simulink model "silnikDC_bezwladnosc_fuzzy"  (R2013b)
settings: Solver=ode3  StartTime=0.0  StopTime=1  FixedStep=100e-6  MaxStep=0.0001  RelTol=1e-3
values from neighbouring files (symbols this model uses):
  a = 0.7    [parametryDC.m]
  B = 0.002953    [parametryDC.m]
  J = 0.02215    [parametryDC.m]
  K = 1.28    [parametryDC.m]
  k1 = 1.28    [parametryDC.m]
  La = 0.1215    [parametryDC.m]
  Ra = 11.2    [parametryDC.m]
  w_de = 1/100000    (= 1e-05)    [parametryDC.m]
  w_du = 100000    [parametryDC.m]
  w_e = 1/2000    (= 0.0005)    [parametryDC.m]
  w_u = 800    [parametryDC.m]
libraries: fuzblock x3
settings Model: Creator=Siembab  LastModifiedBy=Siembab
settings SolverCC: ZeroCrossAlgorithm=Adaptive
settings DataIOCC: SignalLoggingSaveFormat=ModelDataLogs
settings OptimizationCC: ExpressionDepthLimit=2147483647
settings DebuggingCC: FcnCallInpInsideContextMsg=UseLocalSettings  StateNameClashWarn=warning
settings GRTTargetCC: CombineOutputUpdateFcns=off  GRTInterface=on

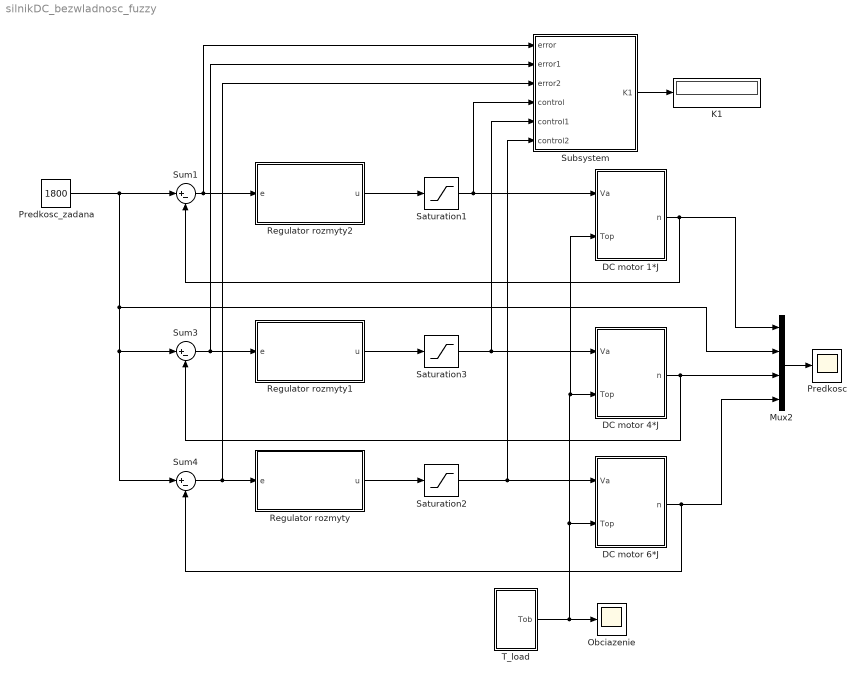
== system silnikDC_bezwladnosc_fuzzy ==
  DC motor 1*J : Subsystem
  DC motor 4*J : Subsystem
  DC motor 6*J : Subsystem
  K1 : Display
  Mux2 : Mux
  Obciazenie : Scope
      settings: TimeRange=1  YMin=1400  YMax=1825
  Predkosc : Scope
      settings: TimeRange=1  YMin=1475  YMax=1825  SaveName=ScopeData4
  Predkosc_zadana : Constant  Value=1800
  Regulator rozmyty : Subsystem
  Regulator rozmyty1 : Subsystem
  Regulator rozmyty2 : Subsystem
  Saturation1 : Saturate  UpperLimit=500  LowerLimit=-500
  Saturation2 : Saturate  UpperLimit=500  LowerLimit=-500
  Saturation3 : Saturate  UpperLimit=500  LowerLimit=-500
  Subsystem : Subsystem
  Sum1 : Sum  Inputs=|+-
  Sum3 : Sum  Inputs=|+-
  Sum4 : Sum  Inputs=|+-
  T_load : Subsystem
  wires:
  Saturation1/1 -> Subsystem/4(control), DC motor 1*J/1(Va)
  Predkosc_zadana/1 -> Sum4/1, Sum3/1, Mux2/2, Sum1/1
  DC motor 1*J/1(n) -> Sum1/2, Mux2/1
  Mux2/1 -> Predkosc/1
  DC motor 6*J/1(n) -> Sum4/2, Mux2/4
  DC motor 4*J/1(n) -> Sum3/2, Mux2/3
  Regulator rozmyty/1(u) -> Saturation2/1
  Saturation2/1 -> Subsystem/6(control2), DC motor 6*J/1(Va)
  Regulator rozmyty1/1(u) -> Saturation3/1
  Saturation3/1 -> Subsystem/5(control1), DC motor 4*J/1(Va)
  Sum3/1 -> Subsystem/2(error1), Regulator rozmyty1/1(e)
  Sum4/1 -> Subsystem/3(error2), Regulator rozmyty/1(e)
  Regulator rozmyty2/1(u) -> Saturation1/1
  Sum1/1 -> Subsystem/1(error), Regulator rozmyty2/1(e)
  T_load/1(Tob) -> Obciazenie/1, DC motor 1*J/2(Top), DC motor 4*J/2(Top), DC motor 6*J/2(Top)
  Subsystem/1(K1) -> K1/1

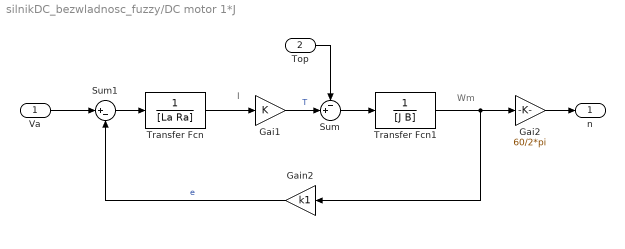
== system silnikDC_bezwladnosc_fuzzy/DC motor 1*J ==
  note: Wm
  note: I
  Va : Inport
  Top : Inport  Port=2
  Gai1 : Gain  Gain=K
  Gai2 : Gain  Gain=60/2*pi
  Gain2 : Gain  Gain=k1
  Sum : Sum  Inputs=-+|
  Sum1 : Sum  Inputs=|+-
  Transfer Fcn : TransferFcn  Denominator=[La Ra]
  Transfer Fcn1 : TransferFcn  Denominator=[J B]
  n : Outport
  wires:
  Transfer Fcn/1 -> Gai1/1
  Gai1/1 -> Sum/2  "T"
  Sum/1 -> Transfer Fcn1/1
  Gain2/1 -> Sum1/2  "e"
  Transfer Fcn1/1 -> Gai2/1, Gain2/1
  Sum1/1 -> Transfer Fcn/1
  Va/1 -> Sum1/1
  Top/1 -> Sum/1
  Gai2/1 -> n/1

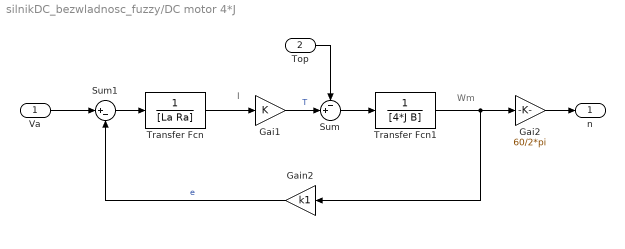
== system silnikDC_bezwladnosc_fuzzy/DC motor 4*J ==
  note: Wm
  note: I
  Va : Inport
  Top : Inport  Port=2
  Gai1 : Gain  Gain=K
  Gai2 : Gain  Gain=60/2*pi
  Gain2 : Gain  Gain=k1
  Sum : Sum  Inputs=-+|
  Sum1 : Sum  Inputs=|+-
  Transfer Fcn : TransferFcn  Denominator=[La Ra]
  Transfer Fcn1 : TransferFcn  Denominator=[4*J B]
  n : Outport
  wires:
  Transfer Fcn/1 -> Gai1/1
  Gai1/1 -> Sum/2  "T"
  Sum/1 -> Transfer Fcn1/1
  Gain2/1 -> Sum1/2  "e"
  Transfer Fcn1/1 -> Gai2/1, Gain2/1
  Sum1/1 -> Transfer Fcn/1
  Va/1 -> Sum1/1
  Top/1 -> Sum/1
  Gai2/1 -> n/1

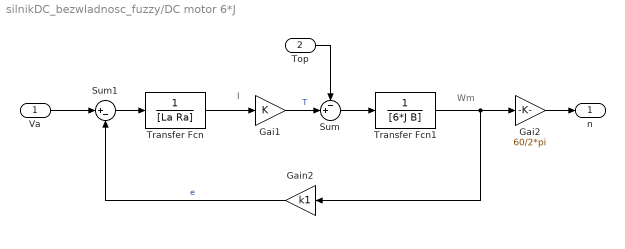
== system silnikDC_bezwladnosc_fuzzy/DC motor 6*J ==
  note: Wm
  note: I
  Va : Inport
  Top : Inport  Port=2
  Gai1 : Gain  Gain=K
  Gai2 : Gain  Gain=60/2*pi
  Gain2 : Gain  Gain=k1
  Sum : Sum  Inputs=-+|
  Sum1 : Sum  Inputs=|+-
  Transfer Fcn : TransferFcn  Denominator=[La Ra]
  Transfer Fcn1 : TransferFcn  Denominator=[6*J B]
  n : Outport
  wires:
  Transfer Fcn/1 -> Gai1/1
  Gai1/1 -> Sum/2  "T"
  Sum/1 -> Transfer Fcn1/1
  Gain2/1 -> Sum1/2  "e"
  Transfer Fcn1/1 -> Gai2/1, Gain2/1
  Sum1/1 -> Transfer Fcn/1
  Va/1 -> Sum1/1
  Top/1 -> Sum/1
  Gai2/1 -> n/1

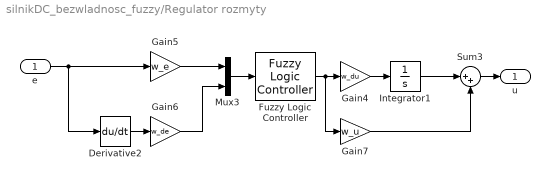
== system silnikDC_bezwladnosc_fuzzy/Regulator rozmyty ==
  e : Inport
  Derivative2 : Derivative
  Fuzzy Logic Controller : fuzblock/Fuzzy Logic  Controller  fis=RegMamdani2
  Gain4 : Gain  Gain=w_du
  Gain5 : Gain  Gain=w_e
  Gain6 : Gain  Gain=w_de
  Gain7 : Gain  Gain=w_u
  Integrator1 : Integrator
  Mux3 : Mux  Inputs=2
  Sum3 : Sum  Inputs=|++
  u : Outport
  wires:
  Derivative2/1 -> Gain6/1
  e/1 -> Derivative2/1, Gain5/1
  Sum3/1 -> u/1
  Gain6/1 -> Mux3/2
  Gain5/1 -> Mux3/1
  Gain7/1 -> Sum3/2
  Mux3/1 -> Fuzzy Logic Controller/1
  Integrator1/1 -> Sum3/1
  Gain4/1 -> Integrator1/1
  Fuzzy Logic Controller/1 -> Gain7/1, Gain4/1

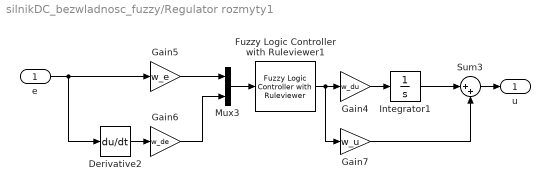
== system silnikDC_bezwladnosc_fuzzy/Regulator rozmyty1 ==
  e : Inport
  Derivative2 : Derivative
  Fuzzy Logic Controller with Ruleviewer1 : fuzblock/Fuzzy Logic  Controller  with Ruleviewer  fismatrix=RegMamdani2  Ts=0.02
  Gain4 : Gain  Gain=w_du
  Gain5 : Gain  Gain=w_e
  Gain6 : Gain  Gain=w_de
  Gain7 : Gain  Gain=w_u
  Integrator1 : Integrator
  Mux3 : Mux  Inputs=2
  Sum3 : Sum  Inputs=|++
  u : Outport
  wires:
  Derivative2/1 -> Gain6/1
  e/1 -> Derivative2/1, Gain5/1
  Sum3/1 -> u/1
  Gain6/1 -> Mux3/2
  Gain5/1 -> Mux3/1
  Gain7/1 -> Sum3/2
  Mux3/1 -> Fuzzy Logic Controller with Ruleviewer1/1
  Integrator1/1 -> Sum3/1
  Gain4/1 -> Integrator1/1
  Fuzzy Logic Controller with Ruleviewer1/1 -> Gain7/1, Gain4/1

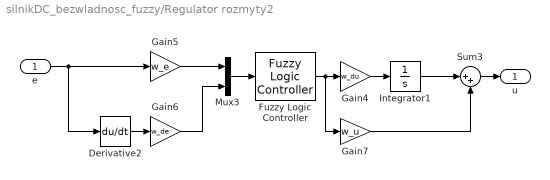
== system silnikDC_bezwladnosc_fuzzy/Regulator rozmyty2 ==
  e : Inport
  Derivative2 : Derivative
  Fuzzy Logic Controller : fuzblock/Fuzzy Logic  Controller  fis=RegMamdani2
  Gain4 : Gain  Gain=w_du
  Gain5 : Gain  Gain=w_e
  Gain6 : Gain  Gain=w_de
  Gain7 : Gain  Gain=w_u
  Integrator1 : Integrator
  Mux3 : Mux  Inputs=2
  Sum3 : Sum  Inputs=|++
  u : Outport
  wires:
  Derivative2/1 -> Gain6/1
  e/1 -> Derivative2/1, Gain5/1
  Sum3/1 -> u/1
  Gain6/1 -> Mux3/2
  Gain5/1 -> Mux3/1
  Gain7/1 -> Sum3/2
  Mux3/1 -> Fuzzy Logic Controller/1
  Integrator1/1 -> Sum3/1
  Gain4/1 -> Integrator1/1
  Fuzzy Logic Controller/1 -> Gain7/1, Gain4/1

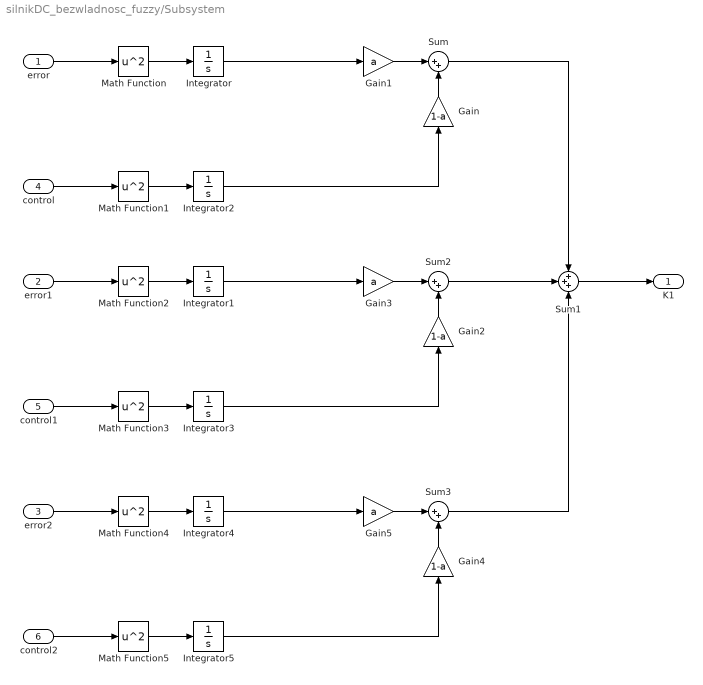
== system silnikDC_bezwladnosc_fuzzy/Subsystem ==
  error : Inport
  error1 : Inport  Port=2
  error2 : Inport  Port=3
  control : Inport  Port=4
  control1 : Inport  Port=5
  control2 : Inport  Port=6
  Gain : Gain  Gain=1-a
  Gain1 : Gain  Gain=a
  Gain2 : Gain  Gain=1-a
  Gain3 : Gain  Gain=a
  Gain4 : Gain  Gain=1-a
  Gain5 : Gain  Gain=a
  Integrator{,1..5} (6 alike) : Integrator
  Math Function{,1..5} (6 alike) : Math  Operator=square  SaturateOnIntegerOverflow=on
  Sum : Sum  Inputs=|++
  Sum1 : Sum  Inputs=+++
  Sum2 : Sum  Inputs=|++
  Sum3 : Sum  Inputs=|++
  K1 : Outport
  wires:
  Integrator2/1 -> Gain/1
  Math Function1/1 -> Integrator2/1
  Gain/1 -> Sum/2
  Gain1/1 -> Sum/1
  Math Function/1 -> Integrator/1
  Integrator/1 -> Gain1/1
  error/1 -> Math Function/1
  control/1 -> Math Function1/1
  Integrator3/1 -> Gain2/1
  Math Function3/1 -> Integrator3/1
  Gain2/1 -> Sum2/2
  Gain3/1 -> Sum2/1
  Math Function2/1 -> Integrator1/1
  Integrator1/1 -> Gain3/1
  error1/1 -> Math Function2/1
  control1/1 -> Math Function3/1
  Integrator5/1 -> Gain4/1
  Math Function5/1 -> Integrator5/1
  Gain4/1 -> Sum3/2
  Gain5/1 -> Sum3/1
  Math Function4/1 -> Integrator4/1
  Integrator4/1 -> Gain5/1
  error2/1 -> Math Function4/1
  control2/1 -> Math Function5/1
  Sum2/1 -> Sum1/2
  Sum3/1 -> Sum1/3
  Sum/1 -> Sum1/1
  Sum1/1 -> K1/1

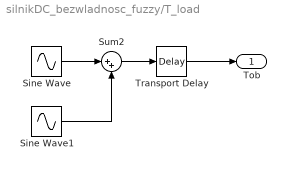
== system silnikDC_bezwladnosc_fuzzy/T_load ==
  Sine Wave : Sin  Amplitude=8  Bias=10  Frequency=100  SampleTime=0
  Sine Wave1 : Sin  Amplitude=8/3  Bias=10  Frequency=3*100  SampleTime=0
  Sum2 : Sum  Inputs=|++
  Transport Delay : TransportDelay  DelayTime=0.5
  Tob : Outport
  wires:
  Sum2/1 -> Transport Delay/1
  Transport Delay/1 -> Tob/1
  Sine Wave1/1 -> Sum2/2
  Sine Wave/1 -> Sum2/1
